simulink model "untitled1"  (R2022b)
settings: Solver=VariableStepAuto  StartTime=0.0  StopTime=10.0  RelTol=1e-3
settings Model: Creator=86157  LastModifiedBy=86157

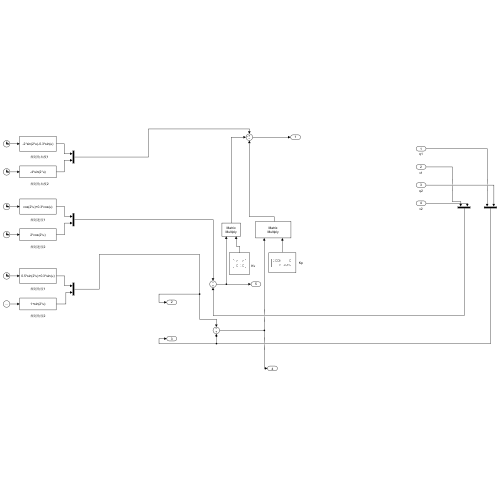
[thumbnail: Simulink's stored preview of the top-level diagram]
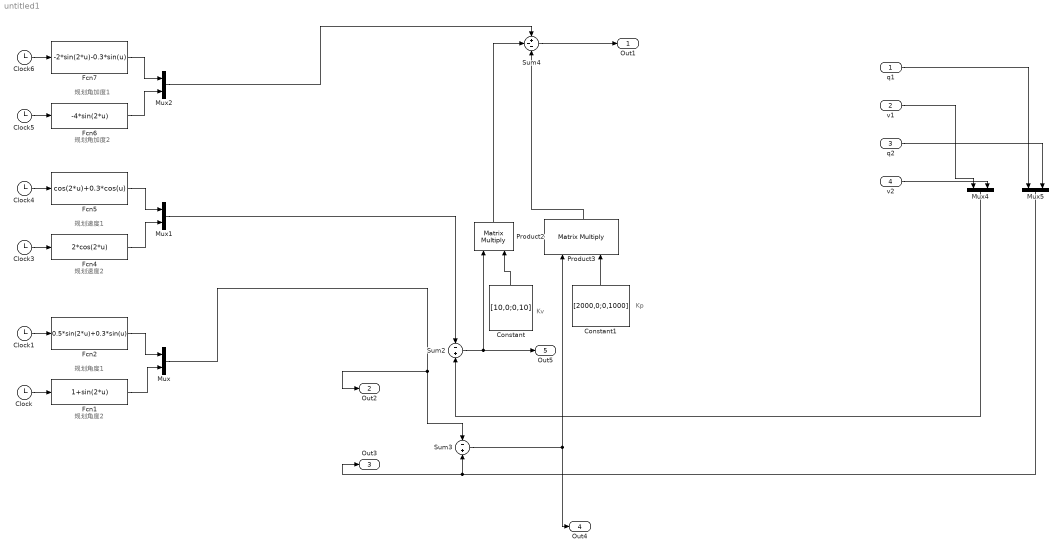
== system untitled1 ==
  note: 规划角度2
  note: 规划角度1
  note: 规划速度1
  note: Kv
  note: 规划角加度1
  note: 规划速度2
  note: 规划角加度2
  note: Kp
  q1 : Inport
  v1 : Inport  Port=2
  q2 : Inport  Port=3
  v2 : Inport  Port=4
  Clock{,1,3..6} (6 alike) : Clock
  Constant : Constant  Value=[10,0;0,10]  VectorParams1D=off
  Constant1 : Constant  Value=[2000,0;0,1000]  VectorParams1D=off
  Fcn1 : Fcn  Expr=1+sin(2*u)
  Fcn2 : Fcn  Expr=0.5*sin(2*u)+0.3*sin(u)
  Fcn4 : Fcn  Expr=2*cos(2*u)
  Fcn5 : Fcn  Expr=cos(2*u)+0.3*cos(u)
  Fcn6 : Fcn  Expr=-4*sin(2*u)
  Fcn7 : Fcn  Expr=-2*sin(2*u)-0.3*sin(u)
  Mux{,1..2,4..5} (5 alike) : Mux  Inputs=2
  Product2 : Product  Multiplication=Matrix(*)
  Product3 : Product  Multiplication=Matrix(*)
  Sum2 : Sum  Inputs=-+
  Sum3 : Sum  Inputs=-+
  Sum4 : Sum  Inputs=+--
  Out1 : Outport
  Out2 : Outport  Port=2
  Out3 : Outport  Port=3
  Out4 : Outport  Port=4
  Out5 : Outport  Port=5
  wires:
  Sum4/1 -> Out1/1
  Sum3/1 -> Product3/1, Out4/1
  Product2/1 -> Sum4/2
  Constant/1 -> Product2/2
  Mux4/1 -> Sum2/2
  v2/1 -> Mux4/2
  Product3/1 -> Sum4/3
  v1/1 -> Mux4/1
  q2/1 -> Mux5/2
  Mux5/1 -> Out3/1, Sum3/2
  Constant1/1 -> Product3/2
  Fcn1/1 -> Mux/2
  Clock1/1 -> Fcn2/1
  Sum2/1 -> Out5/1, Product2/1
  Fcn4/1 -> Mux1/2
  Fcn7/1 -> Mux2/1
  Mux1/1 -> Sum2/1
  Fcn2/1 -> Mux/1
  Clock4/1 -> Fcn5/1
  Fcn6/1 -> Mux2/2
  Fcn5/1 -> Mux1/1
  Clock5/1 -> Fcn6/1
  q1/1 -> Mux5/1
  Clock3/1 -> Fcn4/1
  Mux/1 -> Out2/1, Sum3/1
  Clock/1 -> Fcn1/1
  Clock6/1 -> Fcn7/1
  Mux2/1 -> Sum4/1
